simulink model "FK"  (R2021a)
settings: Solver=VariableStepAuto  StartTime=0.0  StopTime=10.0  RelTol=1e-3
undefined symbols (not defined in the file or in its folder): eul2tform, trvec2tform
libraries: robotcorelib x3, robotmaniplib x2
settings Model: Creator=loris  LastModifiedBy=angelo

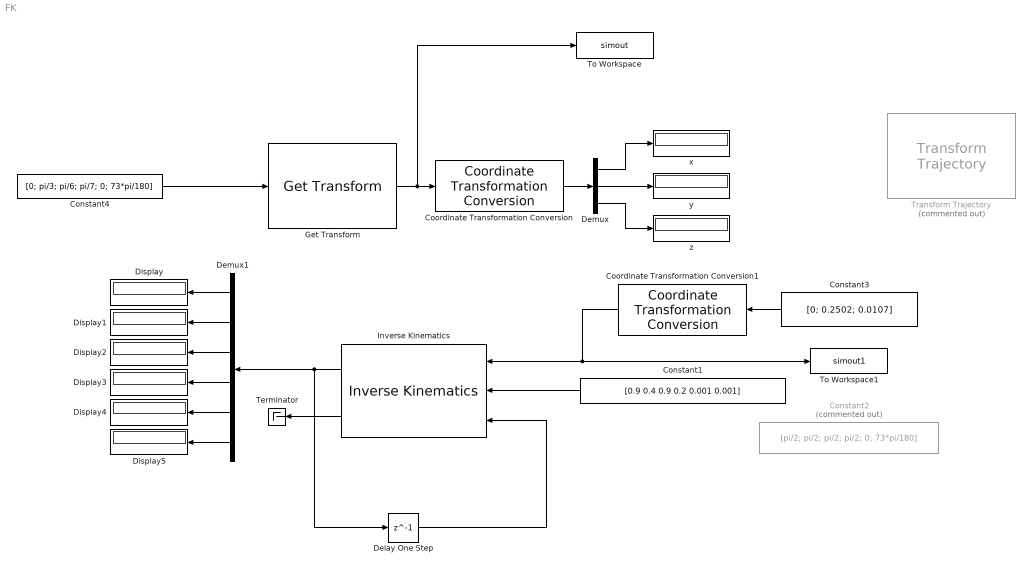
== system FK ==
  Constant1 : Constant  Value=[0.9 0.4 0.9 0.2 0.001 0.001]  VectorParams1D=off
  Constant2 : Constant  Commented=on  Value=[pi/2; pi/2; pi/2; pi/2; 0; 73*pi/180]
  Constant3 : Constant  Value=[0; 0.2502; 0.0107]
  Constant4 : Constant  Value=[0; pi/3; pi/6; pi/7; 0; 73*pi/180]
  Coordinate Transformation Conversion : robotcorelib/Coordinate Transformation Conversion  InputRepresentation=Homogeneous Transformation  InputEulerSequence=ZYX  ShowTrVecInputPort=on  OutputRepresentation=Translation Vector  OutputEulerSequence=ZYX  ShowTrVecOutputPort=on  SimulateUsing=Code generation
      settings: SourceProductBaseCode=NV,RO,RR,UV
  Coordinate Transformation Conversion1 : robotcorelib/Coordinate Transformation Conversion  InputRepresentation=Translation Vector  InputEulerSequence=ZYX  ShowTrVecInputPort=on  OutputRepresentation=Homogeneous Transformation  OutputEulerSequence=ZYX  ShowTrVecOutputPort=on  SimulateUsing=Interpreted execution
      settings: SourceProductBaseCode=NV,RO,RR,UV
  Delay One Step : Delay  DelayLength=1  InputProcessing=Columns as channels (frame based)
  Demux : Demux  Outputs=3
  Demux1 : Demux  Outputs=6
  Display{,1..5} (6 alike) : Display
  Get Transform : robotmaniplib/Get Transform  RigidBodyTree=oRbtRobot  SourceBody=ee  TargetBody=base_link  SimulateUsing=Interpreted execution
  Inverse Kinematics : robotmaniplib/Inverse Kinematics  RigidBodyTree=oRbtRobot  EndEffector=ee  ShowInfo=on  SolverName=BFGS Gradient Projection  EnforceJointLimits=on  MaxIterations=1500  MaxTime=10  GradientTolerance=1e-7  SolutionTolerance=1e-6  StepTolerance=1e-14  ErrorChangeTolerance=1e-12  UseErrorDamping=on  DampingBias=0.0025  SimulateUsing=Interpreted execution
  Terminator : Terminator
  To Workspace : ToWorkspace  VariableName=simout  SaveFormat=Structure  SampleTime=-1
  To Workspace1 : ToWorkspace  VariableName=simout1  SaveFormat=Structure  SampleTime=-1
  Transform Trajectory : robotcorelib/Transform Trajectory  Commented=on  WaypointSource=Internal  T0=trvec2tform( [ 1, 10, -1 ] )  TF=eul2tform( [ 0, pi, pi / 2 ] )  TimeInterval=[ 2, 3 ]  CustomTimeScaling=off  ParameterSource=Internal  TSTime=2:0.1:3  TimeScaling=[ 0:0.1:1; ones( 1, 11 ); zeros( 1, 11 ) ]  SimulateUsing=Interpreted execution
      settings: SourceProductBaseCode=NV,RO,RR,UV
  x : Display
  y : Display
  z : Display
  wires:
  Get Transform/1 -> To Workspace/1, Coordinate Transformation Conversion/1
  Coordinate Transformation Conversion/1 -> Demux/1
  Demux/1 -> x/1
  Demux/2 -> y/1
  Demux/3 -> z/1
  Constant1/1 -> Inverse Kinematics/2
  Inverse Kinematics/1 -> Demux1/1, Delay One Step/1
  Inverse Kinematics/2 -> Terminator/1
  Demux1/1 -> Display/1
  Demux1/2 -> Display1/1
  Demux1/3 -> Display2/1
  Demux1/4 -> Display3/1
  Demux1/5 -> Display4/1
  Demux1/6 -> Display5/1
  Constant3/1 -> Coordinate Transformation Conversion1/1
  Coordinate Transformation Conversion1/1 -> Inverse Kinematics/1, To Workspace1/1
  Delay One Step/1 -> Inverse Kinematics/3
  Constant4/1 -> Get Transform/1
